simulink model "PD_Controller"  (R2019a)
settings: Solver=VariableStepAuto  StartTime=0.0  StopTime=50  RelTol=1e-3
undefined symbols (not defined in the file): G1, G2
settings Model: Creator=Gabe Casciano  LastModifiedBy=Gabe Casciano

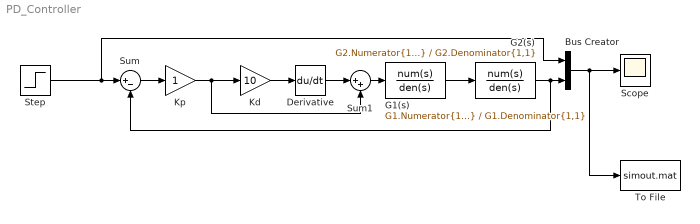
== system PD_Controller ==
  Bus Creator : BusCreator  Inputs=2
  Derivative : Derivative
  G1(s) : TransferFcn  Numerator=G1.Numerator{1,1}  Denominator=G1.Denominator{1,1}
  G2(s) : TransferFcn  Numerator=G2.Numerator{1,1}  Denominator=G2.Denominator{1,1}
  Kd : Gain  Gain=10
  Kp : Gain
  Scope : Scope
  Step : Step  SampleTime=0
  Sum : Sum  Inputs=|+-
  Sum1 : Sum  Inputs=|++
  To File : ToFile  Filename=simout.mat  SaveFormat=Timeseries
  wires:
  Kd/1 -> Derivative/1
  Derivative/1 -> Sum1/1
  Bus Creator/1 -> To File/1, Scope/1
  Sum/1 -> Kp/1
  Step/1 -> Bus Creator/1, Sum/1
  G1(s)/1 -> G2(s)/1
  G2(s)/1 -> Sum/2, Bus Creator/2
  Kp/1 -> Sum1/2, Kd/1
  Sum1/1 -> G1(s)/1
